simulink model "part4simulation_starterBUTitsforpart6"  (R2024b)
settings: Solver=ode5  StartTime=0.0  StopTime=7  FixedStep=.002  MaxStep=.001  RelTol=1e-3
undefined symbols (not defined in the file): Adwn, Aup, B, C, L_newdwn, L_newup
settings Model: Creator=d-block  LastModifiedBy=fve2

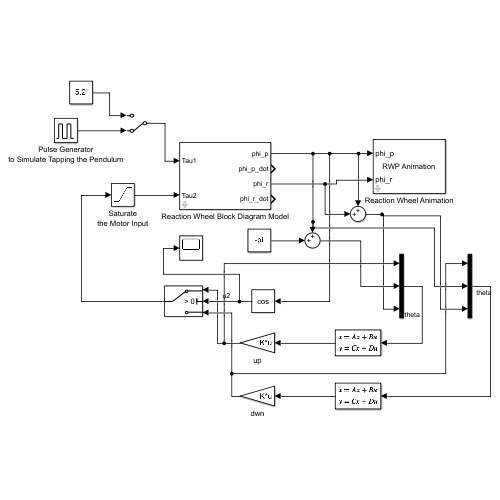
[thumbnail: Simulink's stored preview of the top-level diagram]
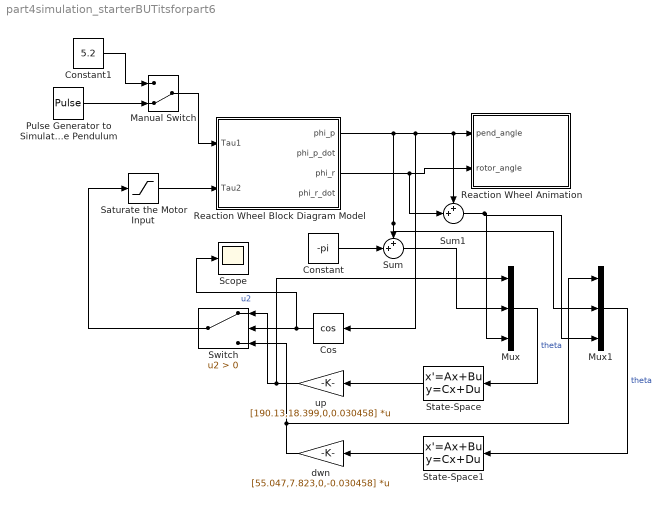
== system part4simulation_starterBUTitsforpart6 ==
  Constant : Constant  Value=-pi
  Constant1 : Constant  Value=5.2
  Cos : Trigonometry  Operator=cos
  Manual Switch : ManualSwitch  CurrentSetting=0
  Mux : Mux  Inputs=3
  Mux1 : Mux  Inputs=3
  Pulse Generator to Simulate Tapping the Pendulum : DiscretePulseGenerator  PulseType=Time based  Amplitude=0  Period=4  PulseWidth=5
  Reaction Wheel Animation : Subsystem  mask(Reaction Wheel Animation){}
      mask help: The animation block takes as input the pendulum angle (in radians), with 0 pointing down. Use this to visualize the pendulum position while testing controllers.
      mask Help: The animation block takes as input the pendulum angle (in radians), with 0 pointing down.  Use this to visualize the pendulum position while testing controllers.
      mask Display:
      | port_label('input', 1, 'phi_p')
      | port_label('input', 2, 'phi_r')
      | fprintf('RWP Animation')
  Reaction Wheel Block Diagram Model : Subsystem  mask(Reaction Wheel Block Diagram Model){par=[78.4 1.08 198], g=9.804, init=[pi/12 1 0 0]}
      mask prompts: par "Internal Parameters (a, bp, br)"; g "Acceleration of Gravity"; init "Initial Conditions"
      mask help:
      | This is a <i>nonlinear mathematical model</i> of the reaction wheel pendulum.  It takes as inputs torques to the system, and outputs a state vector.
      | <p>
      | <h2>Parameters</h2>
      | <ul>
      | <h3>Internal Parameters</h3>
      | <ul>
      | <li><b>a</b>, the square of the frquency of small oscillations ( a = omega<sub>p</sub><sup>2</sup>) </li>
      | <li><b>b<sub>p</sub></b>, the control gain over total inertia (b<sub>p</sub> = k<sub>u</sub>/J)</li>
      | <li><b>b<sub>r</sub></b>, the control gain over rotor inertia (b<sub>r</sub> = k<sub>u</sub>/J<sub>r</sub>)</li>
      | </ul>
      | <h3>Acceleration of Gravity</h3>
      | <ul>
      | <li><b>g</b>, commonly 9.804</li>
      | </ul>
      | <h3>Initial Conditions</h3>
      | Starting values for the state vector.  Usually, use [pi, 0,0,0] to start the pendulum at rest in the unstable equilibrium position pointing upwards.
      | <ul>
      | <li><b>phi<sub>p</sub></b>, encoder angle of the pendulum, in radians (0 is down)</li>
      | <li><b>phi<sub>p</sub>dot</b>, angular velocity of the pendulum, in radians/sec</li>
      | <li><b>phi<sub>r</sub></b>, encoder angle of the rotor, in radians (0 is down)</li>
      | <li><b>phi<sub>r</sub>dot</b>, angular velocity of the pendulum, in radians/sec</li>
      | </ul>
      | </ul>
      | <p>
      mask Help:
      | This is a <i>nonlinear mathematical model</i>  of the reaction wheel pendulum.  It takes as inputs torques to the system, and outputs a state vector.
      | <p>
      | <h2>Parameters</h2>
      | <ul>
      | <h3>Internal Parameters</h3>
      | <ul>
      | <li><b>a</b>, the square of the frquency of small oscillations ( a = omega<sub>p</sub><sup>2</sup>) </li>
      | <li><b>b<sub>p</sub></b>, the control gain over total inertia (b<sub>p</sub> = k<sub>u</sub>/J)</li>
      | <li><b>b<sub>r</sub></b>, the control gain over rotor inertia (b<sub>r</sub> = k<sub>u</sub>/J<sub>r</sub>)</li>
      | </ul>
      | <h3>Acceleration of Gravity</h3>
      | <ul>
      | <li><b>g</b>, commonly 9.804</li>
      | </ul>
      | <h3>Initial Conditions</h3>
      | Starting values for the state vector.  Usually, use [pi, 0,0,0] to start the pendulum at rest in the unstable equilibrium position pointing upwards.
      | <ul>
      | <li><b>phi<sub>p</sub></b>, encoder angle of the pendulum, in radians (0 is down)</li>
      | <li><b>phi<sub>p</sub>dot</b>, angular velocity of the pendulum, in radians/sec</li>
      | <li><b>phi<sub>r</sub></b>, encoder angle of the rotor, in radians (0 is down)</li>
      | <li><b>phi<sub>r</sub>dot</b>, angular velocity of the pendulum, in radians/sec</li>
      | </ul>
      | </ul>
      | <p>
      | 
      | <h2>Inputs</h2>
      | <ul>
      | <li><b>Tau1</b>, external force on the pendulum arm. (This arm is not actuated, but disturbances can be applied here)</li>
      | <li><b>Tau2</b>, external force on the rotor.  (input to the motor + disturbances)</li>
      | </ul>
      | 
      | <h2>Outputs</h2>
      | <ul>
      |  Outputs the current state vector. (See Initial Conditions)
      | </ul>
      | <p>
      | Don’t forget to include a Saturation block (to saturate the control effort at +/- 10) before <i>Tau2</i>.
      | <p>
      | <!-- last updates, Summer, 2007 -->
  Saturate the Motor Input : Saturate  UpperLimit=10  LowerLimit=-10
  Scope : Scope
  State-Space : StateSpace  A=Aup-L_newup*C  B=[B L_newup]  C=eye(4)  D=zeros(4,3)  InitialCondition=0
  State-Space1 : StateSpace  A=Adwn-L_newdwn*C  B=[B L_newdwn]  C=eye(4)  D=zeros(4,3)  InitialCondition=0
  Sum : Sum  Inputs=++|
  Sum1 : Sum  Inputs=++|
  Switch : Switch  Criteria=u2 > Threshold  SaturateOnIntegerOverflow=off  InputSameDT=off
  dwn : Gain  Gain=[55.047,7.823,0,-0.030458]  Multiplication=Matrix(K*u)
  up : Gain  Gain=[190.13,18.399,0,0.030458]  Multiplication=Matrix(K*u)
  wires:
  Reaction Wheel Block Diagram Model/1(phi_p) -> Mux1/2, Sum/1, Cos/1, Sum1/1, Reaction Wheel Animation/1(pend_angle)
  Reaction Wheel Block Diagram Model/3(phi_r) -> Sum1/2, Reaction Wheel Animation/2(rotor_angle)
  Saturate the Motor Input/1 -> Reaction Wheel Block Diagram Model/2(Tau2)
  Constant1/1 -> Manual Switch/1
  Pulse Generator to Simulate Tapping the Pendulum/1 -> Manual Switch/2
  Manual Switch/1 -> Reaction Wheel Block Diagram Model/1(Tau1)
  Mux/1 -> State-Space/1  "theta"
  State-Space/1 -> up/1
  Constant/1 -> Sum/2
  Sum/1 -> Mux/2
  Sum1/1 -> Mux1/3, Mux/3
  Cos/1 -> Scope/1, Switch/2  "u2"
  Switch/1 -> Saturate the Motor Input/1
  dwn/1 -> Mux1/1, Switch/3
  up/1 -> Mux/1, Switch/1
  State-Space1/1 -> dwn/1
  Mux1/1 -> State-Space1/1  "theta"

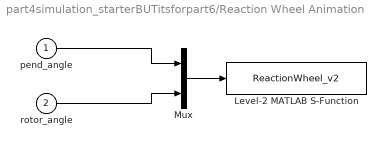
== system part4simulation_starterBUTitsforpart6/Reaction Wheel Animation ==
  pend_angle : Inport
  rotor_angle : Inport  Port=2
  Level-2 MATLAB S-Function : M-S-Function  FunctionName=ReactionWheel_v2
  Mux : Mux  Inputs=2
  wires:
  pend_angle/1 -> Mux/1
  rotor_angle/1 -> Mux/2
  Mux/1 -> Level-2 MATLAB S-Function/1

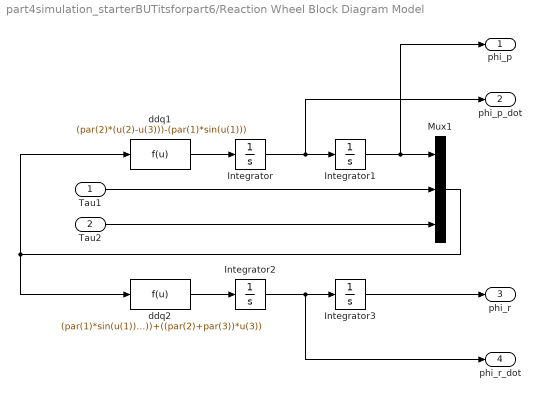
== system part4simulation_starterBUTitsforpart6/Reaction Wheel Block Diagram Model ==
  Tau1 : Inport
  Tau2 : Inport  Port=2
  Integrator : Integrator  InitialCondition=init(2)
  Integrator1 : Integrator  InitialCondition=init(1)
  Integrator2 : Integrator  InitialCondition=init(4)
  Integrator3 : Integrator  InitialCondition=init(3)
  Mux1 : Mux  Inputs=3
  ddq1 : Fcn  Expr=(par(2)*(u(2)-u(3)))-(par(1)*sin(u(1)))
  ddq2 : Fcn  Expr=(par(1)*sin(u(1)))-(par(2)*u(2))+((par(2)+par(3))*u(3))
  phi_p : Outport
  phi_p_dot : Outport  Port=2
  phi_r : Outport  Port=3
  phi_r_dot : Outport  Port=4
  wires:
  ddq1/1 -> Integrator/1
  ddq2/1 -> Integrator2/1
  Integrator3/1 -> phi_r/1
  Integrator2/1 -> phi_r_dot/1, Integrator3/1
  Integrator/1 -> phi_p_dot/1, Integrator1/1
  Integrator1/1 -> phi_p/1, Mux1/1
  Tau1/1 -> Mux1/2
  Tau2/1 -> Mux1/3
  Mux1/1 -> ddq2/1, ddq1/1
